simulink library "tres_simulink_blockset"  (R2014a)
settings: Solver=ode45  StartTime=0.0  StopTime=10.0  RelTol=1e-3
settings Model: Creator=matteo  LastModifiedBy=matteo

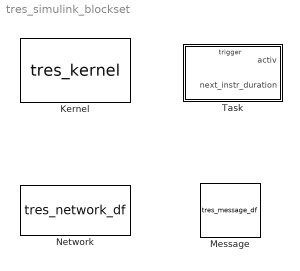
== system tres_simulink_blockset ==
  Kernel : S-Function  FunctionName=tres_kernel  Parameters=taskset_descr_name scheduling_policy sched_pol_descr dead_miss_rule time_res core_num under_engine  EnableBusSupport=off  mask{taskset_descr_name=, scheduling_policy=DEADLINE_MONOTONIC, sched_pol_descr=, dead_miss_rule=Continue, time_res=Milli_Seconds, core_num=1, under_engine=RTSIM}
      mask prompts: taskset_descr_name "Task-Set Description"; scheduling_policy "Scheduling Policy"; sched_pol_descr "Scheduling Policy Description"; dead_miss_rule "Deadline-Miss Handling"; time_res "Time Resolution"; core_num "Number of CPU Cores"; under_engine "Engine"
      mask Callback taskset_descr_name: kernel_tsdescr_cb(gcb)
      mask TypeOptions scheduling_policy: DEADLINE_MONOTONIC | EDF | FIXED_PRIORITY | OTHER
      mask Callback scheduling_policy: kernel_schedpolicy_cb(gcb)
      mask Callback sched_pol_descr: kernel_scheddescr_cb(gcb)
      mask TypeOptions dead_miss_rule: Continue | Kill Instance
      mask TypeOptions time_res: Seconds | Milli_Seconds | Micro_Seconds | Nano_Seconds
      mask Callback core_num: kernel_coreno_cb(gcb)
      mask TypeOptions under_engine: RTSIM
      mask Display:
      | port_label('output', 1, 'activ')
      | port_label('input', 1, 'duration')
      | port_label('input', 2, 'trigger')
  Message : S-Function  FunctionName=tres_message_df  Parameters=num_msg_objects  EnableBusSupport=off  mask{num_msg_objects=1}
      mask prompts: num_msg_objects "Number of Application Level Message Objects"
      mask Callback num_msg_objects: message_nummsgobjs_cb(gcb)
      mask Display:
      | port_label('input', 1, 'wake')
      | port_label('output', 1, 'activ')
  Network : S-Function  FunctionName=tres_network_df  Parameters=msgset_descr_name time_res under_engine net_descr_name other_deps  EnableBusSupport=off  mask{msgset_descr_name=, time_res=Micro_Seconds, under_engine=OMNeT++, net_descr_name=, other_deps=[]}
      mask prompts: msgset_descr_name "Message-Set Description"; time_res "Time Resolution"; under_engine "Engine"; net_descr_name "Network Description (Simulation-Specific)"; other_deps "Additional Libraries (Simulation-Specific)"
      mask Callback msgset_descr_name: network_msgdescr_cb(gcb)
      mask TypeOptions time_res: Seconds | Milli_Seconds | Micro_Seconds | Nano_Seconds
      mask TypeOptions under_engine: OMNeT++
      mask Callback net_descr_name: network_netdescr_cb(gcb)
      mask Callback other_deps: network_otherdeps_cb(gcb)
      mask Display: port_label('output', 1, 'activ')
  Task : Subsystem  TreatAsAtomicUnit=on  mask{conf_name=}
      mask prompts: conf_name "Name of the Configuration Variable"
      mask init:
      | set_param(sprintf('%s/Task',gcb),'Parameters','conf_name')
      mask Callback conf_name: task_instrdescr_cb(gcb)

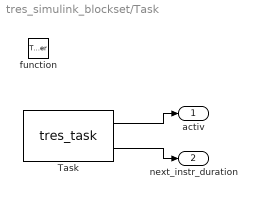
== system tres_simulink_blockset/Task ==
  function : TriggerPort  TriggerType=function-call
  Task : S-Function  FunctionName=tres_task  Parameters=conf_name  EnableBusSupport=off
  activ : Outport
  next_instr_duration : Outport  Port=2
  wires:
  Task/1 -> activ/1
  Task/2 -> next_instr_duration/1
